simulink model "manifold_matlab"  (R2022b)
settings: Solver=ode45  StartTime=0.0  StopTime=10.0  MaxStep=0.2  RelTol=1e-3  EnableMultiTasking=on
InitFcn:
  | % Input data
  | load manifold_press_start.mat
settings Model: Creator=dlange  LastModifiedBy=bensweet
settings SolverCC: AlgebraicLoopSolver=TrustRegion
settings DataIOCC: ExternalInput=[t, mdot_in, w]  LimitDataPoints=on  LoadExternalInput=on  SaveFormat=Array  ReturnWorkspaceOutputs=off
settings OptimizationCC: ExpressionDepthLimit=2147483647  InitFltsAndDblsToZero=on  LifeSpan=inf
settings DebuggingCC: UnconnectedInputMsg=warning  UnconnectedOutputMsg=warning  UnconnectedLineMsg=warning  PregeneratedLibrarySubsystemCodeDiagnostic=none  SFMachineParentedDataDiag=warning
settings HardwareCC: ProdBitPerPointer=32  ProdBitPerSizeT=32  ProdBitPerPtrDiffT=32  ProdLargestAtomicFloat=None  ProdIntDivRoundTo=Undefined  ProdEndianess=Unspecified  ProdWordSize=32  ProdHWDeviceType=32-bit Generic
settings ModelReferenceCC: EnableRefExpFcnMdlSchedulingChecks=on  PropagateSignalLabelsOutOfModel=off
settings SFSimCC: SimUseLocalCustomCode=off  SimParseCustomCode=off
settings RTWCC: RTWUseLocalCustomCode=off  DLArmComputeVersion=19.05
settings CodeAppCC: StateflowObjectComments=on
settings GRTTargetCC: TargetFcnLib=ansi_tfl_tmw.mat  TargetLangStandard=C89/C90 (ANSI)  CombineOutputUpdateFcns=off  GRTInterface=on
settings ConfigComp: CovMetricSettings=dw  CovSaveCumulativeToWorkspaceVar=on  CovSaveSingleToWorkspaceVar=on  CovExternalEMLEnable=off  CovSFcnEnable=off

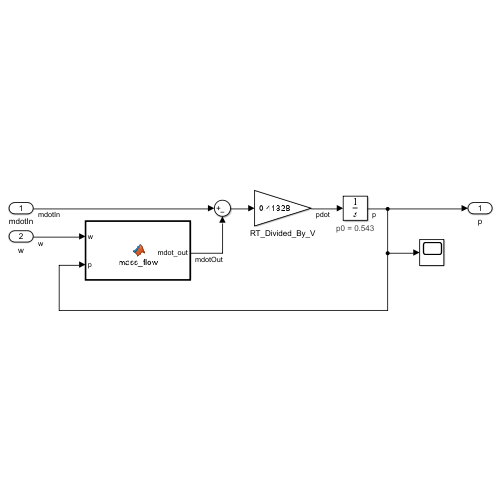
[thumbnail: Simulink's stored preview of the top-level diagram]
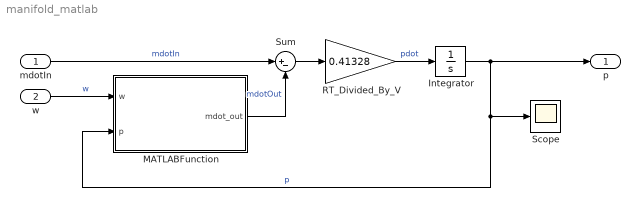
== system manifold_matlab ==
  mdotIn : Inport
  w : Inport  Port=2
  Integrator : Integrator  InitialCondition=0.543
      settings: AttributesFormatString=p0 = %<InitialCondition>
  MATLABFunction : MATLAB Function  TreatAsAtomicUnit=on
  RT_Divided_By_V : Gain  Gain=0.41328
  Scope : Scope
  Sum : Sum  Inputs=|+-
  p : Outport  VectorParamsAs1DForOutWhenUnconnected=off
  wires:
  Integrator/1 -> p/1, MATLABFunction/2(p), Scope/1  "p"
  RT_Divided_By_V/1 -> Integrator/1  "pdot"
  mdotIn/1 -> Sum/1  "mdotIn"
  Sum/1 -> RT_Divided_By_V/1
  w/1 -> MATLABFunction/1(w)  "w"
  MATLABFunction/1(mdot_out) -> Sum/2  "mdotOut"

== matlab function manifold_matlab/MATLABFunction ==
  data: w input; mdot_out output; p input
function mdot_out = mass_flow(w,p)
% This block uses MATLAB language features supported for
% code generation. See the help menu for details. 

mdot_out = -0.366 + 0.08979*w*p - 0.0337*w*p^2 + 0.0001*w^2*p;
